simulink library "EarthPointing"  (R2014b)
settings: Solver=ode45  SolverMode=SingleTasking  StartTime=0.0  StopTime=10.0  RelTol=1e-3
undefined symbols (not defined in the file or in its folder): confEstim, ConfParam
libraries: Qprod x2, Mat2Quat x2, Normalization x2, CrossProd x2, Qinverse x1, Quat2Rot x1, TransformMatrix x1
settings Model: Creator=y.akisheva  LastModifiedBy=Hp
settings OptimizationCC: BlockReduction=off  BooleanDataType=off  UseDivisionForNetSlopeComputation=off  SimCompilerOptimization=off
settings DebuggingCC: SaveWithParameterizedLinksMsg=none  UnderspecifiedInitializationDetection=Classic  MergeDetectMultiDrivingBlocksExec=none  SignalResolutionControl=TryResolveAllWithWarning  SolverPrmCheckMsg=none  FrameProcessingCompatibilityMsg=error  AllowSymbolicDim=off  StrictBusMsg=Warning
settings HardwareCC: TargetUnknown=on
settings RTWCC: RTWCompilerOptimization=off
settings ConfigComp: CovMetricSettings=dw  CovHtmlReporting=on  CovSaveCumulativeToWorkspaceVar=on  CovSaveSingleToWorkspaceVar=on  CovModelRefEnable=Off  CovExternalEMLEnable=off  CovSFcnEnable=off

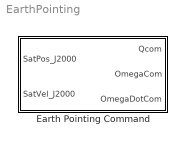
== system EarthPointing ==
  Earth Pointing Command : Subsystem

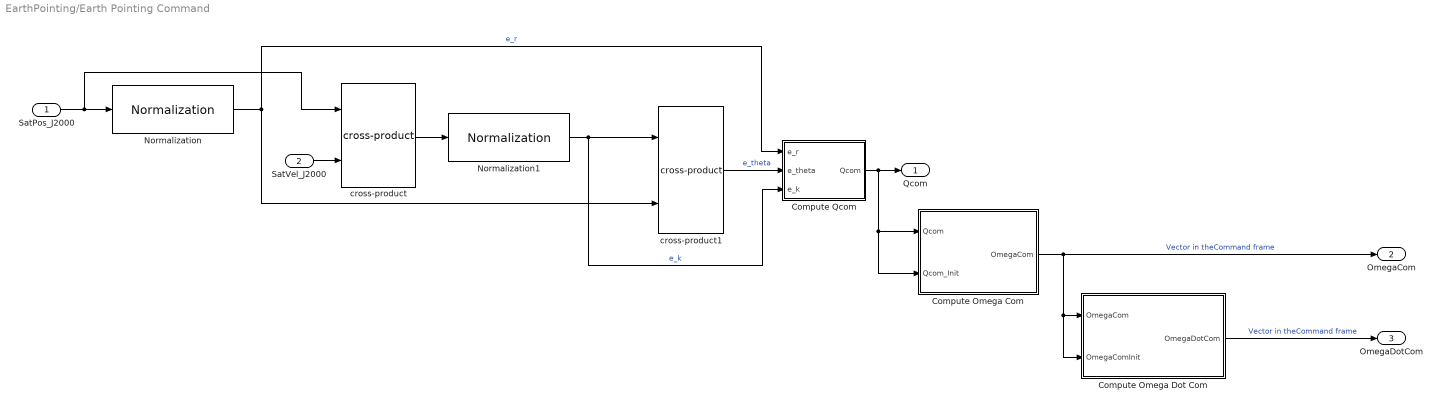
== system EarthPointing/Earth Pointing Command ==
  SatPos_J2000 : Inport
  SatVel_J2000 : Inport  Port=2
  Compute Omega Com : Subsystem
  Compute Omega Dot Com : Subsystem
  Compute Qcom : Subsystem
  Normalization : Normalization/Normalization
  Normalization1 : Normalization/Normalization
  cross-product : CrossProd/cross-product
  cross-product1 : CrossProd/cross-product
  Qcom : Outport
  OmegaCom : Outport  Port=2
  OmegaDotCom : Outport  Port=3
  wires:
  Normalization/1 -> cross-product1/2, Compute Qcom/1(e_r)  "e_r"
  SatVel_J2000/1 -> cross-product/2
  cross-product/1 -> Normalization1/1
  SatPos_J2000/1 -> Normalization/1, cross-product/1
  Normalization1/1 -> Compute Qcom/3(e_k), cross-product1/1  "e_k"
  Compute Omega Dot Com/1(OmegaDotCom) -> OmegaDotCom/1  "Vector in theCommand frame"
  Compute Omega Com/1(OmegaCom) -> OmegaCom/1, Compute Omega Dot Com/2(OmegaComInit), Compute Omega Dot Com/1(OmegaCom)  "Vector in theCommand frame"
  Compute Qcom/1(Qcom) -> Compute Omega Com/2(Qcom_Init), Compute Omega Com/1(Qcom), Qcom/1
  cross-product1/1 -> Compute Qcom/2(e_theta)  "e_theta"

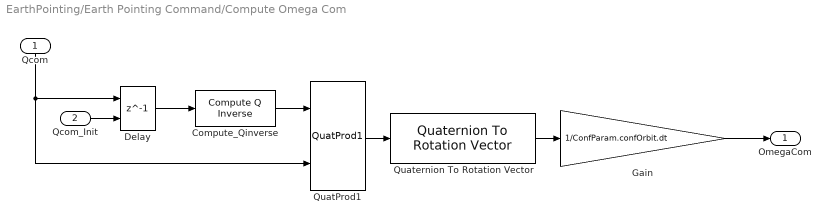
== system EarthPointing/Earth Pointing Command/Compute Omega Com ==
  Qcom : Inport
  Qcom_Init : Inport  Port=2
  Compute_Qinverse : Qinverse/Compute Q Inverse
  Delay : Delay  DelayLength=1  InitialConditionSource=Input port  InitialCondition=confEstim.InitQsat  SampleTime=ConfParam.confOrbit.dt
      settings: InputPortMap=u0,p4
  Gain : Gain  Gain=1/ConfParam.confOrbit.dt
  QuatProd1 : Qprod/QuatProd1
  Quaternion To Rotation Vector : Quat2Rot/Quaternion To Rotation Vector
  OmegaCom : Outport
  wires:
  Qcom/1 -> QuatProd1/2, Delay/1
  Quaternion To Rotation Vector/1 -> Gain/1
  Gain/1 -> OmegaCom/1
  QuatProd1/1 -> Quaternion To Rotation Vector/1
  Delay/1 -> Compute_Qinverse/1
  Qcom_Init/1 -> Delay/2
  Compute_Qinverse/1 -> QuatProd1/1

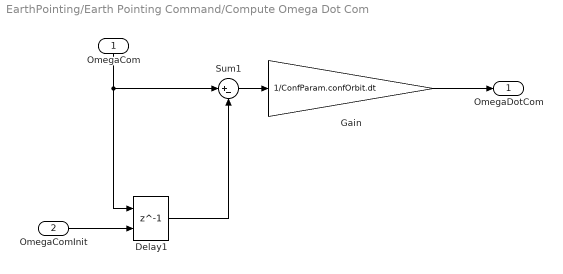
== system EarthPointing/Earth Pointing Command/Compute Omega Dot Com ==
  OmegaCom : Inport
  OmegaComInit : Inport  Port=2
  Delay1 : Delay  DelayLength=1  InitialConditionSource=Input port  InitialCondition=confEstim.InitQsat  SampleTime=ConfParam.confOrbit.dt
      settings: InputPortMap=u0,p4
  Gain : Gain  Gain=1/ConfParam.confOrbit.dt
  Sum1 : Sum  Inputs=|+-
  OmegaDotCom : Outport
  wires:
  OmegaCom/1 -> Sum1/1, Delay1/1
  Gain/1 -> OmegaDotCom/1
  Sum1/1 -> Gain/1
  OmegaComInit/1 -> Delay1/2
  Delay1/1 -> Sum1/2

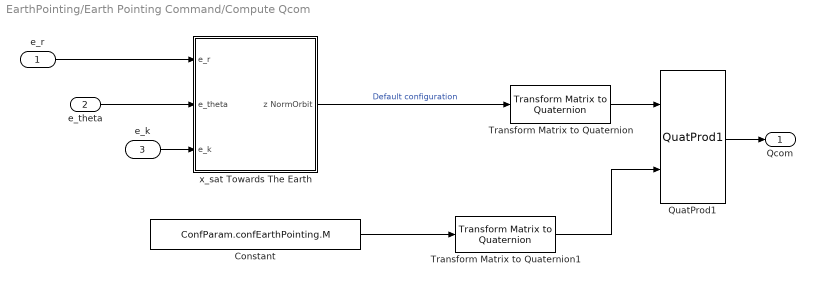
== system EarthPointing/Earth Pointing Command/Compute Qcom ==
  e_r : Inport
  e_theta : Inport  Port=2
  e_k : Inport  Port=3
  Constant : Constant  Value=ConfParam.confEarthPointing.M
  QuatProd1 : Qprod/QuatProd1
  Transform Matrix to Quaternion : Mat2Quat/Transform Matrix to Quaternion
  Transform Matrix to Quaternion1 : Mat2Quat/Transform Matrix to Quaternion
  x_sat Towards The Earth : Subsystem
  Qcom : Outport
  wires:
  e_r/1 -> x_sat Towards The Earth/1(e_r)
  e_k/1 -> x_sat Towards The Earth/3(e_k)
  Transform Matrix to Quaternion/1 -> QuatProd1/1
  e_theta/1 -> x_sat Towards The Earth/2(e_theta)
  x_sat Towards The Earth/1(z NormOrbit) -> Transform Matrix to Quaternion/1  "Default configuration"
  Transform Matrix to Quaternion1/1 -> QuatProd1/2
  QuatProd1/1 -> Qcom/1
  Constant/1 -> Transform Matrix to Quaternion1/1

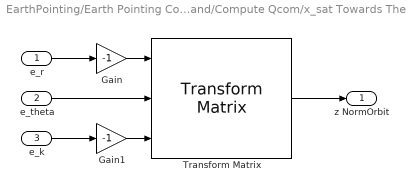
== system EarthPointing/Earth Pointing Command/Compute Qcom/x_sat Towards The Earth ==
  e_r : Inport
  e_theta : Inport  Port=2
  e_k : Inport  Port=3
  Gain : Gain  Gain=-1
  Gain1 : Gain  Gain=-1
  Transform Matrix : TransformMatrix/Transform Matrix
  z NormOrbit : Outport
  wires:
  e_theta/1 -> Transform Matrix/2
  e_k/1 -> Gain1/1
  e_r/1 -> Gain/1
  Gain/1 -> Transform Matrix/1
  Transform Matrix/1 -> z NormOrbit/1
  Gain1/1 -> Transform Matrix/3
